simulink library "Average"  (Simulink 8.2)
settings: Solver=ode45  StartTime=0.0  StopTime=10.0  RelTol=1e-3
settings Model: Creator=lena.frank  LastModifiedBy=drhf

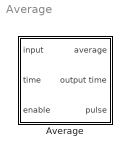
== system Average ==
  Average : Subsystem  mask{time_intervall=1 h, offset_flag=on, enable_flag=on}
      mask prompts: time_intervall "Delta t"; offset_flag "start calculating every full hour"; enable_flag "only calculate when enabled"
      mask help:
      | This block calculates the average of each input vector during a specified time Delta_t. During this time interval the output is held.
      | The output time is the time of the last average calculation.
      |  Every time the average is calculated again, a signal pulse of 1 is put out.
      |
      | When the full hour flag is set, the calculation of the average is started every full hour once again.
      |
      | When the enable flag is set, the functions calculates only while the enable signal is 1. When it is 0, the function repeats putting out the last output.
      mask init:
      | time_list = [3600 1800 900 600 300];
      | delta_t = time_list(time_intervall);
      mask Help: web(fullfile(path_carnot('help'),'Average.html'),'-helpbrowser')
      mask TypeOptions time_intervall: 1 h | 30 min | 15 min | 10 min | 5 min

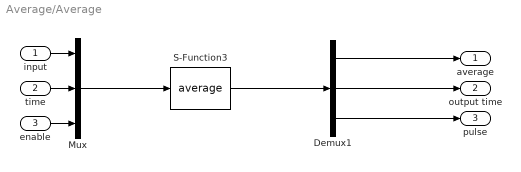
== system Average/Average ==
  input : Inport
  time : Inport  Port=2
  enable : Inport  Port=3
  Demux1 : Demux  Outputs=[-1 1 1]
  Mux : Mux  Inputs=3
  S-Function3 : S-Function  FunctionName=average  Parameters=delta_t offset_flag enable_flag  EnableBusSupport=off
  average : Outport
  output time : Outport  Port=2
  pulse : Outport  Port=3
  wires:
  Demux1/3 -> pulse/1
  Demux1/2 -> output time/1
  Demux1/1 -> average/1
  enable/1 -> Mux/3
  time/1 -> Mux/2
  input/1 -> Mux/1
  S-Function3/1 -> Demux1/1
  Mux/1 -> S-Function3/1
